simulink model "Bai5A_4"  (R2015a)
settings: Solver=ode45  StartTime=0.0  StopTime=10.0  RelTol=1e-3
libraries: commchan3 x1, dsparch4 x1, commsink2 x1, commutil2 x1, commfilt2 x1, dspstat3 x1, commrandsrc2 x1
settings Model: Creator=Trong  LastModifiedBy=Trong

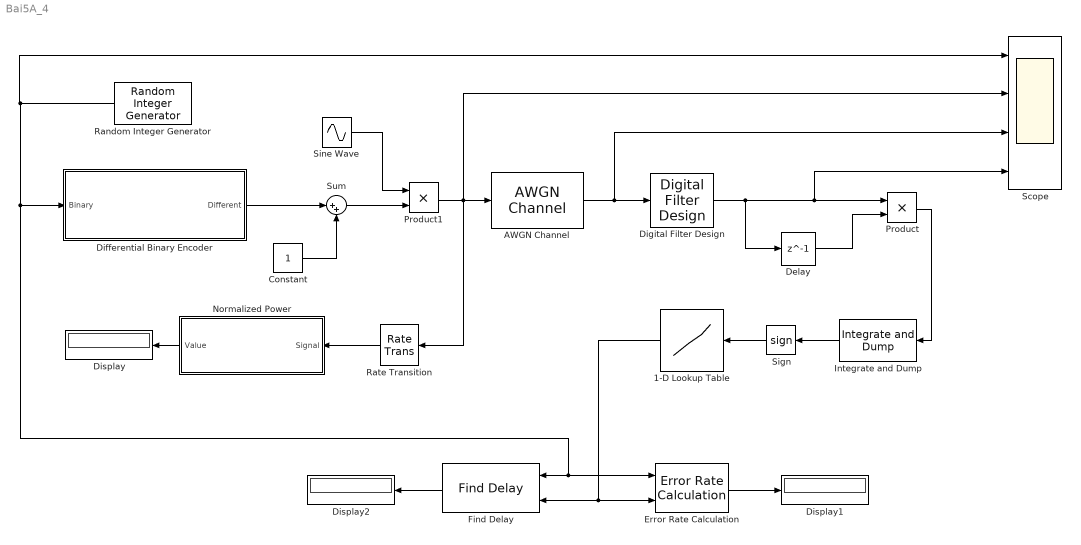
== system Bai5A_4 ==
  1-D Lookup Table : Lookup_n-D  NumberOfTableDimensions=1  BreakpointsForDimension1=[-5:5]  Table=tanh([-5:5])  InternalRulePriority=Speed  RndMeth=Simplest  InputSameDT=on
  AWGN Channel : commchan3/AWGN Channel  InputProcessing=Columns as channels (frame based)  seed=67  noiseMode="Signal to noise ratio  (Eb/No)"  EbNodB=10  EsNodB=10  SNRdB=10  bitsPerSym=1  Ps=1  Tsym=1  variance=1
  Constant : Constant
  Delay : Delay  DelayLength=1  InitialCondition=0
  Differential Binary Encoder : Subsystem
  Digital Filter Design : dsparch4/Digital Filter Design  mwdsp_browser_bugfix_var=off
  Display : Display
  Display1 : Display
  Display2 : Display
  Error Rate Calculation : commsink2/Error Rate Calculation  N=0  st_delay=0  cp_mode=Entire frame  subframe=[]  PMode=Port  WsName=ErrorVec  RsMode2=off  stop=off  numErr=100  maxBits=1e6
  Find Delay : commutil2/Find Delay  corrLength=200  chgSigOP=off  stopUpdate=off  numConstDelay=3
  Integrate and Dump : commfilt2/Integrate and Dump  obssamples=8  offsetsamples=0  nodump=off  roundingMode=Floor  overflowMode=off
  Normalized Power : Subsystem
  Product : Product
  Product1 : Product
  Random Integer Generator : commrandsrc2/Random Integer Generator  mul=8  seed=37  Ts=1  frameBased=off  sampPerFrame=1  orient=off  outDataType=double
  Rate Transition : RateTransition
  Scope : Scope  NumInputPorts=4
      settings: YMin=-5~-5~-5~-5  YMax=5~5~5~5
  Sign : Signum
  Sine Wave : Sin  SampleTime=0
  Sum : Sum  Inputs=|++
  wires:
  Differential Binary Encoder/1(Different) -> Sum/1
  Constant/1 -> Sum/2
  AWGN Channel/1 -> Scope/3, Digital Filter Design/1
  Product1/1 -> Rate Transition/1, Scope/2, AWGN Channel/1
  Sum/1 -> Product1/2
  Sine Wave/1 -> Product1/1
  Digital Filter Design/1 -> Delay/1, Scope/4, Product/1
  Delay/1 -> Product/2
  Product/1 -> Integrate and Dump/1
  Integrate and Dump/1 -> Sign/1
  Sign/1 -> 1-D Lookup Table/1
  Normalized Power/1(Value) -> Display/1
  Rate Transition/1 -> Normalized Power/1(Signal)
  Error Rate Calculation/1 -> Display1/1
  1-D Lookup Table/1 -> Error Rate Calculation/2, Find Delay/2
  Random Integer Generator/1 -> Error Rate Calculation/1, Find Delay/1, Differential Binary Encoder/1(Binary), Scope/1
  Find Delay/1 -> Display2/1

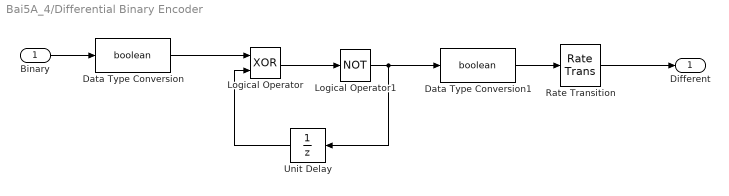
== system Bai5A_4/Differential Binary Encoder ==
  Binary : Inport
  Data Type Conversion : DataTypeConversion  OutDataTypeStr=boolean
  Data Type Conversion1 : DataTypeConversion  OutDataTypeStr=boolean
  Logical Operator : Logic  Operator=XOR  AllPortsSameDT=off  OutDataTypeStr=boolean
  Logical Operator1 : Logic  Operator=NOT  AllPortsSameDT=off  OutDataTypeStr=boolean
  Rate Transition : RateTransition
  Unit Delay : UnitDelay  SampleTime=-1
  Different : Outport
  wires:
  Binary/1 -> Data Type Conversion/1
  Logical Operator1/1 -> Data Type Conversion1/1, Unit Delay/1
  Rate Transition/1 -> Different/1
  Logical Operator/1 -> Logical Operator1/1
  Unit Delay/1 -> Logical Operator/2
  Data Type Conversion1/1 -> Rate Transition/1
  Data Type Conversion/1 -> Logical Operator/1

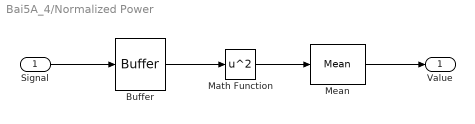
== system Bai5A_4/Normalized Power ==
  Signal : Inport
  Buffer : Buffer  TreatMby1Signals=One channel
  Math Function : Math  Operator=square  SaturateOnIntegerOverflow=on
  Mean : dspstat3/Mean  run=off  reset_popup=None  InputProcessing=Columns as channels (frame based)  directionMode=Each column  dimension=1  treatSBRowAsCol=off  roiEnable=off  roiType=Rectangles  roiPortion=Entire ROI  roiOutput=Individual statistics for each ROI  roiFlag=off  outputDataTypeStr=Inherit: Same as accumulator  outputLastDataTypeStr=Inherit: Same as accumulator  outputMin=[]  outputMax=[]  roundingMode=Floor  overflowMode=off
  Value : Outport
  wires:
  Signal/1 -> Buffer/1
  Buffer/1 -> Math Function/1
  Mean/1 -> Value/1
  Math Function/1 -> Mean/1
